simulink model "simple_echo_old"  (R2019a)
settings: Solver=VariableStepAuto  StartTime=0.0  StopTime=10.0  RelTol=1e-3
undefined symbols (not defined in the file or in its folder): a, b, c
libraries: hdlsllib x1
settings Model: Creator=amyel  LastModifiedBy=h34j161

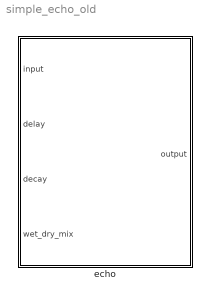
== system simple_echo_old ==
  echo : Subsystem

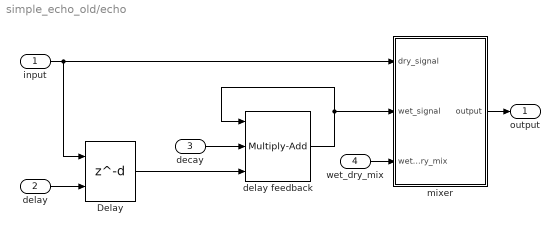
== system simple_echo_old/echo ==
  input : Inport
  delay : Inport  Port=2
  decay : Inport  Port=3
  wet_dry_mix : Inport  Port=4
  Delay : Delay  DelayLengthSource=Input port  DelayLengthUpperLimit=Fs  DiagnosticForDelayLength=Error  UseCircularBuffer=on
      settings: InputPortMap=u0,p1
  delay feedback : hdlsllib/HDL Operations/Multiply-Add  Function=c+(a.*b)  datatype=Inherit: Inherit via internal rule  DoSatur=off  FMA=off
      settings: SourceProductName=Simulink  SourceProductBaseCode=SL
  mixer : Subsystem
  output : Outport
  wires:
  Delay/1 -> delay feedback/3
  delay/1 -> Delay/2
  delay feedback/1 -> mixer/2(wet_signal), delay feedback/1
  input/1 -> mixer/1(dry_signal), Delay/1
  decay/1 -> delay feedback/2
  wet_dry_mix/1 -> mixer/3(wet_dry_mix)
  mixer/1(output) -> output/1

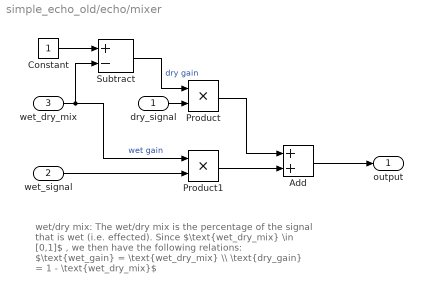
== system simple_echo_old/echo/mixer ==
  note: wet/dry mix:
      | The wet/dry mix is the percentage of the signal that is wet (i.e. effected).
      |
      | Since $\text{wet_dry_mix} \in [0,1]$ , we then have the following relations:
      | $\text{wet_gain} = \text{wet_dry_mix} \\ \text{dry_gain} = 1 - \text{wet_dry_mix}$
  dry_signal : Inport
  wet_signal : Inport  Port=2
  wet_dry_mix : Inport  Port=3
  Add : Sum
  Constant : Constant  SampleTime=-1
  Product : Product
  Product1 : Product
  Subtract : Sum  Inputs=+-
  output : Outport
  wires:
  Add/1 -> output/1
  Constant/1 -> Subtract/1
  wet_dry_mix/1 -> Product1/1, Subtract/2  "wet gain"
  dry_signal/1 -> Product/2
  Subtract/1 -> Product/1  "dry gain"
  Product/1 -> Add/1
  Product1/1 -> Add/2
  wet_signal/1 -> Product1/2
